simulink model "InvertedPendulum_REV2"  (R2018a)
settings: Solver=VariableStepAuto  StartTime=0.0  StopTime=T_STOP  RelTol=1e-3
values from neighbouring files (symbols this model uses):
  A_dist = 0    [InvertedPendulum.m]    (also in InvertedPendulumStepResponse.m)
  Ac = [0 1 0 0 ... (first row only)    [BasicModelParameters.m]    (also in ControllerDesign_REV0.m; FurutaPendulum.m = [0 1 0 0; 0 0 -a23 0; 0 0 0 1; 0 0 a43 0]; InvertedPendulumStepResponse.m)
  Bc = transpose([0 b21 0 -b41])    [BasicModelParameters.m]    (also in ControllerDesign_REV0.m; FurutaPendulum.m = [0; b21; 0; -b41]; InvertedPendulumStepResponse.m)
  Cc = [1 0 0 0 ... (first row only)    [BasicModelParameters.m]    (also in ControllerDesign_REV0.m; FurutaPendulum.m = [1 0 0 0; 0 0 1 0]; InvertedPendulumStepResponse.m)
  Dc = [0 ... (first row only)    [BasicModelParameters.m]    (also in ControllerDesign_REV0.m; FurutaPendulum.m = [0; 0]; InvertedPendulumStepResponse.m)
  f_dist = 10    [InvertedPendulum.m]    (also in InvertedPendulumStepResponse.m)
  k1 = [-5.2947]    [InvertedPendulum.m]    (also in InvertedPendulumStepResponse.m)
  k2 = [-5.1415]    [InvertedPendulum.m]    (also in InvertedPendulumStepResponse.m)
  p1 = [-284.8, 0]    [InvertedPendulum.m]    (also in InvertedPendulumStepResponse.m)
  p2 = [-50]    [InvertedPendulum.m]    (also in InvertedPendulumStepResponse.m)
  Ts = 0.0017    [ControllerDesign_REV0.m]    (also in InvertedPendulum.m; InvertedPendulumStepResponse.m)
  z1 = [-0.1229, -0.02181]    [InvertedPendulum.m]    (also in InvertedPendulumStepResponse.m)
  z2 = [-9.249]    [InvertedPendulum.m]    (also in InvertedPendulumStepResponse.m)
settings Model: Creator=Jack  LastModifiedBy=Jack

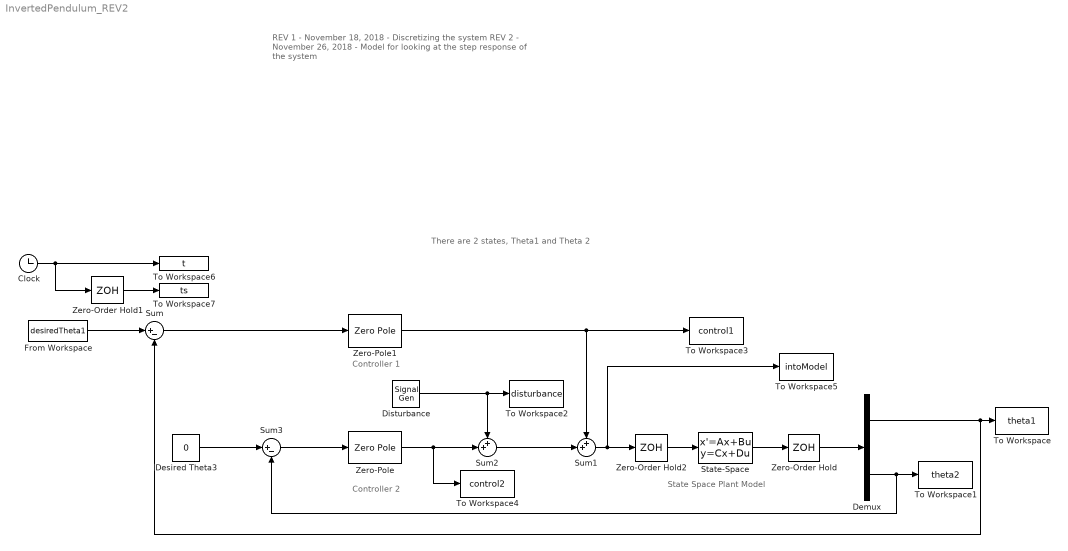
== system InvertedPendulum_REV2 ==
  note: REV 1 -  November 18, 2018
      | 	- Discretizing the system
      | REV 2 - November 26, 2018
      | 	- Model for looking at the step response of the system
  note: Controller 1
  note: There are 2 states, Theta1 and Theta 2
  note: State Space Plant Model
  note: Controller 2
  Clock : Clock
  Demux : Demux  Outputs=2
  Desired Theta3 : Constant  Value=0
  "Disturbance " : SignalGenerator  Amplitude=A_dist  Frequency=f_dist
  From Workspace : FromWorkspace  VariableName=desiredTheta1  SampleTime=0
  State-Space : StateSpace  A=Ac  B=Bc  C=Cc  D=Dc  InitialCondition=[0; 0; 0.05; 0]  ContinuousStateAttributes='Theta'
  Sum : Sum  Inputs=|+-
  Sum1 : Sum  Inputs=++|
  Sum2 : Sum  Inputs=++|
  Sum3 : Sum  Inputs=|+-
  To Workspace : ToWorkspace  VariableName=theta1  SampleTime=-1
  To Workspace1 : ToWorkspace  VariableName=theta2  SampleTime=-1
  To Workspace2 : ToWorkspace  VariableName=disturbance  SampleTime=-1
  To Workspace3 : ToWorkspace  VariableName=control1  SampleTime=-1
  To Workspace4 : ToWorkspace  VariableName=control2  SampleTime=-1
  To Workspace5 : ToWorkspace  VariableName=intoModel  SampleTime=-1
  To Workspace6 : ToWorkspace  VariableName=t  SampleTime=-1
  To Workspace7 : ToWorkspace  VariableName=ts  SampleTime=-1
  Zero-Order Hold : ZeroOrderHold  SampleTime=Ts
  Zero-Order Hold1 : ZeroOrderHold  SampleTime=Ts
  Zero-Order Hold2 : ZeroOrderHold  SampleTime=Ts
  Zero-Pole : ZeroPole  Zeros=z2  Poles=p2  Gain=k2
  Zero-Pole1 : ZeroPole  Zeros=z1  Poles=p1  Gain=k1
  wires:
  From Workspace/1 -> Sum/1
  Sum/1 -> Zero-Pole1/1
  Sum1/1 -> Zero-Order Hold2/1, To Workspace5/1
  Demux/1 -> Sum/2, To Workspace/1
  Demux/2 -> Sum3/2, To Workspace1/1
  Desired Theta3/1 -> Sum3/1
  Zero-Pole/1 -> To Workspace4/1, Sum2/2
  Sum3/1 -> Zero-Pole/1
  "Disturbance "/1 -> Sum2/1, To Workspace2/1
  Sum2/1 -> Sum1/2
  Zero-Pole1/1 -> To Workspace3/1, Sum1/1
  Clock/1 -> Zero-Order Hold1/1, To Workspace6/1
  State-Space/1 -> Zero-Order Hold/1
  Zero-Order Hold/1 -> Demux/1
  Zero-Order Hold1/1 -> To Workspace7/1
  Zero-Order Hold2/1 -> State-Space/1
